simulink model "S_MPPT_CONTROLLERS_SIM_V2"  (R2017a)
settings: Solver=VariableStepAuto  StartTime=0.0  StopTime=11  FixedStep=1e-6  MaxStep=1e-4  RelTol=1e-3
values from neighbouring files (symbols this model uses):
  a = 1    [EXPER_PARAMETERS_V1.m]    (also in M_MPPT_CONTROLLERS_SIM_V1.m; TSUKAMOTO_FUZZY_MODEL_V1.m)
  Cload = 470e-6    (= 0.00047)    [M_MPPT_CONTROLLERS_SIM_V1.m]
  Co = 1e-6    (= 1e-06)    [M_MPPT_CONTROLLERS_SIM_V1.m]
  Dmax = Ucmax    (= 9000)    [EXPER_PARAMETERS_V1.m]    (also in M_MPPT_CONTROLLERS_SIM_V1.m = 65535)
  Fred = fs    (= 60)    [M_MPPT_CONTROLLERS_SIM_V1.m]
  fs = 60    [M_MPPT_CONTROLLERS_SIM_V1.m]
  Icc_calc = In/(5/100)    [M_MPPT_CONTROLLERS_SIM_V1.m]
  K1 = K1y2md    [EXPER_PARAMETERS_V1.m]    (also in M_MPPT_CONTROLLERS_SIM_V1.m = K(1:end-1))
  K2 = Kimd    [EXPER_PARAMETERS_V1.m]    (also in M_MPPT_CONTROLLERS_SIM_V1.m = K(end))
  Kh1 = 1/ipv    (= 0.35)    [EXPER_PARAMETERS_V1.m]    (also in M_MPPT_CONTROLLERS_SIM_V1.m = 0.0636345580933)
  KI1 = Kp1/Ti1*Ts1    (= 760)    [EXPER_PARAMETERS_V1.m]    (also in M_MPPT_CONTROLLERS_SIM_V1.m = 95.322582)
  KI2 = Ki2*Ts4    [M_MPPT_CONTROLLERS_SIM_V1.m]
  KI4 = Ki4*Ts4    [M_MPPT_CONTROLLERS_SIM_V1.m]
  KI5 = Ki5*Ts_inv    (= 0.17765287922)    [M_MPPT_CONTROLLERS_SIM_V1.m]
  KP1 = Kp1-KI1/2    (= 5320)    [EXPER_PARAMETERS_V1.m]    (also in M_MPPT_CONTROLLERS_SIM_V1.m = 4107.638709)
  KP2 = Kp2-KI2/2    [M_MPPT_CONTROLLERS_SIM_V1.m]
  KP4 = Kp4-KI4/2    [M_MPPT_CONTROLLERS_SIM_V1.m]
  KP5 = Kp5*Ts_inv-KI5/2    (= -0.0874937760062)    [M_MPPT_CONTROLLERS_SIM_V1.m]
  L = 4.4e-3    (= 0.0044)    [EXPER_PARAMETERS_V1.m]    (also in M_MPPT_CONTROLLERS_SIM_V1.m = 0.100000049318)
  Linv = 0.0133    [M_MPPT_CONTROLLERS_SIM_V1.m]
  Rinv = 0.0417    [M_MPPT_CONTROLLERS_SIM_V1.m]
  S = 10e3*3/2    (= 15000)    [M_MPPT_CONTROLLERS_SIM_V1.m]
  Ts1 = 1/Fs    (= 0.0002)    [EXPER_PARAMETERS_V1.m]    (also in M_MPPT_CONTROLLERS_SIM_V1.m)
  Ts3 = Ts1    (= 0.0002)    [EXPER_PARAMETERS_V1.m]    (also in M_MPPT_CONTROLLERS_SIM_V1.m; TSUKAMOTO_FUZZY_MODEL_V1.m)
  Ts4 = 1/(4*Fc)    (= 0.000125)    [M_MPPT_CONTROLLERS_SIM_V1.m]
  Ts_inv = 1/(100*Fc)    (= 5e-06)    [M_MPPT_CONTROLLERS_SIM_V1.m]
  Univ_discurso = 0.015*1    (= 0.015)    [EXPER_PARAMETERS_V1.m]    (also in M_MPPT_CONTROLLERS_SIM_V1.m; TSUKAMOTO_FUZZY_MODEL_V1.m)
  vdc = 12    [EXPER_PARAMETERS_V1.m]    (also in M_MPPT_CONTROLLERS_SIM_V1.m = 1000)
  vdc_ref = vdc    (= 12)    [EXPER_PARAMETERS_V1.m]    (also in M_MPPT_CONTROLLERS_SIM_V1.m = 1000)
  Vf = VL/sqrt(3)    [M_MPPT_CONTROLLERS_SIM_V1.m]
  VL = (381.051/2)    (= 190.5255)    [M_MPPT_CONTROLLERS_SIM_V1.m]
undefined symbols (not defined in the file or in its folder): DiscIntNeverNeededParam, sigbuilder_block
undefined symbols (not defined in the file): Fs
libraries: powerlib x22, powerlib_meascontrol x10, fuzblock x4, dsparch4 x3, re_lib x1, simulink x1
(part 2 of 2)

== matlab function S_MPPT_CONTROLLERS_SIM_V2/ DQ control/PID Digital I 3 ==
  data: IN_ref input; UK output; IN input; KI input; KP input
function UK = fcn(IN_ref, IN, KI, KP)

 %Valores iniciales de las conStantes del controlador
 persistent  ek uk
 persistent  ek_1 uk_1
 if isempty(ek)
    ek =0;
    uk =0;
    ek_1 =0;
    uk_1 =0;
 end
ek=IN_ref-IN;
uk=ek*(KP+KI)-ek_1*KP+uk_1;
if(uk>60)
    uk=60;
end
if(uk<-60)
    uk=-60;
end
ek_1=ek;
uk_1=uk;
UK=uk;
end

== matlab function S_MPPT_CONTROLLERS_SIM_V2/PLL/PID Digital I 7 ==
  data: Ref input; Out output; Med input; KI input; KP input
function Out = fcn(Ref, Med, KI, KP)

 %Valores iniciales de las conStantes del controlador
 persistent  ek uk
 persistent  ek_1 uk_1
 if isempty(ek)
    ek =0;
    uk =0;
    ek_1 =0;
    uk_1 =0;
 end
ek=Ref-Med;
%uk=ek*(KP+KI)-ek_1*KP+uk_1;
uk=KP*ek+KI*ek+KI*ek_1;
ek_1=ek;
uk_1=uk;
Out=uk;
end

== matlab function S_MPPT_CONTROLLERS_SIM_V2/Fuzzy Tsukamoto Current Controller n_mppt = 99.11%, ta(2%) = 0.12 s con Steps de Irrad Interv. 2 Seg. n_mppt = 96.74%, ta(2%) = 0.12 s con Steps de Irrad Interv. 0.5 Seg. n_mppt = 99.37%, ta(2%) = 0.12 s con Curva de Irrad Este controlador puede disminuir ta e incrementar a tr para mitigar los MP en id (impacto positivo en PQ) /Linear combination ==
  data: mA1 input; y0 output; mA2 input; Adj input; UD input
function y0 = fcn(mA1,mA2,Adj, UD)
w1=mA1;
w2=mA2;
z1 = -(UD)*(w1-0.5);
z2 = (UD)*(w2-0.5);
y0 = ((w1*z1 + w2*z2)/(w1+w2))+Adj;
end

== matlab function S_MPPT_CONTROLLERS_SIM_V2/Digital State Feedback Current Controller n_mppt = 88.18%, ta(2%) = 0.4 s con Steps de Irrad Interv. 2 Seg. n_mppt = 97.01%, ta(2%) = 0.1 s con Steps de Irrad Interv. 2 Seg. n_mppt = 86.2%, ta(2%) = 0.4 s con Steps de Irrad Interv. 0.5 Seg. n_mppt = 93.3%, ta(2%) = 0.1 s con Steps de Irrad Interv. 0.5 Seg. n_mppt = 96.15%, ta(2%) = 0.1 s con Curva de Irrad ta(2%) de 0.1 s se obtiene el ta de F-Tsukmam n_mppt = 89.31%, ta(2%) = 0.0692 s con Steps de Irrad Interv. 0.5 Seg. Menor ta y tr: mayor n_mppt pero genera mayor MP en id (impacto negativo PQ). Si se mantiene ta y se incrementa tr la n_mppt se mantiene al mismo tiempo que se mitigan los MP en id (impacto positivo en PQ)  /PID Digital I 2 ==
  data: iL_ref input; iL input; UK output; vdc input; KI input; K1 input; K2 input
function UK = fcn(iL_ref, iL, vdc, KI, K1, K2)

 %Valores iniciales de las conStantes del controlador
 persistent  ek Acc_Int uk
 persistent  Acc_Int_1
 if isempty(ek)
    ek =0;
    uk =0;
    Acc_Int =0;
    Acc_Int_1 =0;
 end
ek=iL_ref- iL;
Acc_Int=ek*KI+Acc_Int_1;
Acc_Int_1=Acc_Int;
uk=Acc_Int-(K1*iL+K2*vdc);
if(uk>(1*65535))
    uk=1*65535;
end
if(uk<0)
    uk=0;
end
UK=uk;
end

== matlab function S_MPPT_CONTROLLERS_SIM_V2/A Measurements/n_mppt (%)/MATLAB Function ==
  data: y output; time input
function y = fcn(time)
    % Verifica si el valor es Inf
    if time < 0.201
        y = 1;  % Si es Inf, asigna 0
    else
        y = 0;  % Si no es Inf, devuelve el valor original
    end
end
